simulink model "Bai06_3"  (R2023b)
settings: Solver=VariableStepAuto  StartTime=0.0  StopTime=0.1  RelTol=1e-3
settings Model: Creator=Trung  LastModifiedBy=Trung

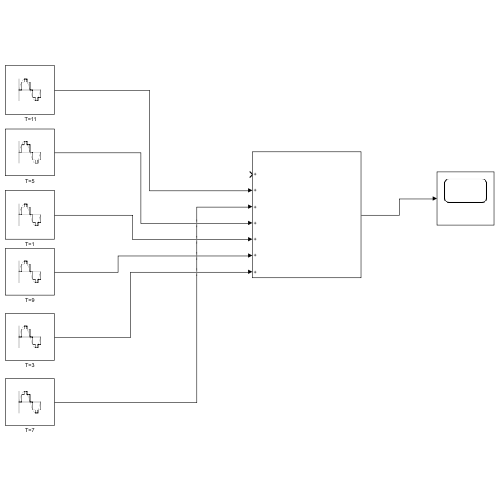
[thumbnail: Simulink's stored preview of the top-level diagram]
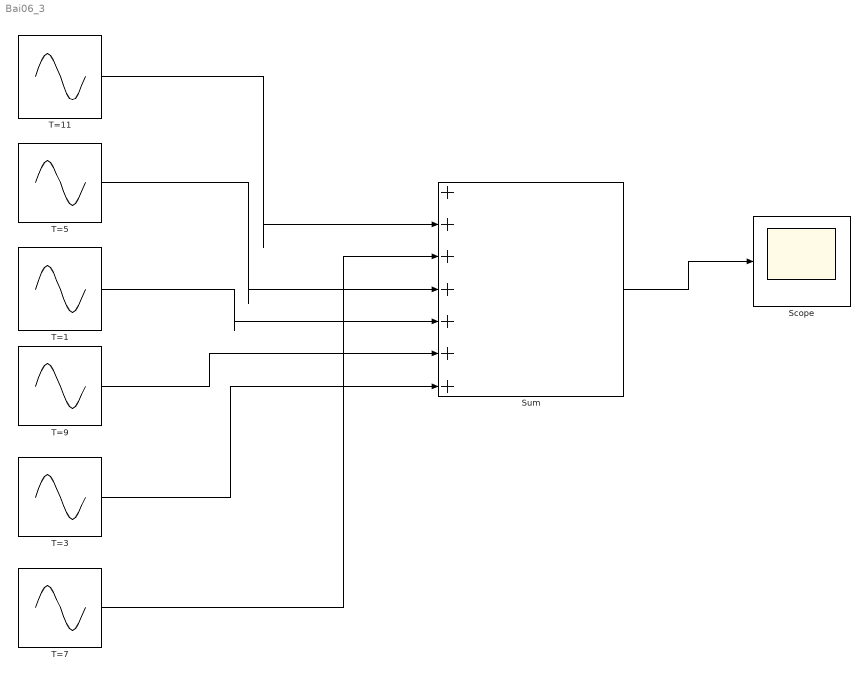
== system Bai06_3 ==
  " T=11" : Sin  Amplitude=1/11  Frequency=50 * pi * 2 * 11  SampleTime=0.0001
  Scope : Scope
  Sum : Sum  Inputs=|+++++++
  T=1 : Sin  Frequency=50 * pi * 2  SampleTime=0.0001
  T=3 : Sin  Amplitude=1/3  Frequency=50*pi*2*3  SampleTime=0.0001
  T=5 : Sin  Amplitude=1/5  Frequency=50*pi*2*5  SampleTime=0.0001
  T=7 : Sin  Amplitude=1/7  Frequency=50*pi*2*7  SampleTime=0.0001
  T=9 : Sin  Amplitude=1/9  Frequency=50*pi*2*9  SampleTime=0.0001
  wires:
  T=5/1 -> Sum/4
  Sum/1 -> Scope/1
  T=3/1 -> Sum/7
  T=1/1 -> Sum/5
  T=7/1 -> Sum/3
  " T=11"/1 -> Sum/2
  T=9/1 -> Sum/6
